simulink model "lo_osc_test"  (Simulink 7.4)
settings: Solver=ode45  StartTime=0.0  StopTime=1000  RelTol=1e-3
libraries: xbsIndex_r4 x8
settings Model: Creator=chenhong  LastModifiedBy=chenhong

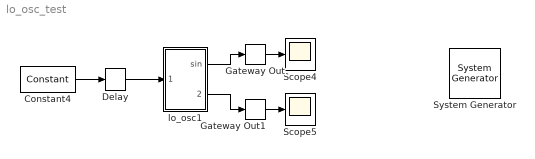
== system lo_osc_test ==
  " System Generator" : xbsIndex_r4/ System Generator  Tag=genX  SystemSampleTime=-1  xilinxfamily=Virtex6  part=xc6vsx315t  speed=-3  package=ff1156  synthesis_tool=XST  clock_wrapper=Clock Enables  directory=./netlist  testbench=off  simulink_period=1  sysclk_period=10  dcm_input_clock_period=10  incr_netlist=off  trim_vbits=Everywhere in SubSystem  dbl_ovrd=According to Block Masks  core_generation=According to Block Masks  run_coregen=off  deprecated_control=off  eval_field=0  block_type=sysgen
      settings: block_version=11.4
  Constant4 : xbsIndex_r4/Constant  arith_type=Boolean  const=1  n_bits=16  bin_pt=14  explicit_period=on  period=1024  equ=P=C  opselect=C  inp2=PCIN>>17  opr=+  inp1=P  carry=CIN  dbl_ovrd=off  block_type=constant
      settings: block_version=11.4
  Delay : xbsIndex_r4/Delay  en=off  latency=25  dbl_ovrd=off  reg_retiming=off  block_type=delay
      settings: block_version=11.4
  Gateway Out : xbsIndex_r4/Gateway Out  hdl_port=on  timing_constraint=None  locs_specified=off  LOCs={}  block_type=gatewayout
      settings: infoedit="Gateway out block.  Converts Xilinx fixed point inputs into ouputs of type Simulink integer, double, or fixed point.<br><br>Hardware notes:  In hardware these blocks become top level output ports or are discarded, depending on how they are configured."  block_version=11.4
  Gateway Out1 : xbsIndex_r4/Gateway Out  hdl_port=on  timing_constraint=None  locs_specified=off  LOCs={}  block_type=gatewayout
      settings: infoedit="Gateway out block.  Converts Xilinx fixed point inputs into ouputs of type Simulink integer, double, or fixed point.<br><br>Hardware notes:  In hardware these blocks become top level output ports or are discarded, depending on how they are configured."  block_version=11.4
  Scope4 : Scope
  Scope5 : Scope
  lo_osc1 : Subsystem  AncestorBlock=xblocks_library_downconverter/lo_osc  mask(lo_osc){n_bits=8, counter_step=5, counter_start=1, counter_width=8, latency=2}
      mask prompts: n_bits "Output Bitwidth"; counter_step "counter step"; counter_start "counter start value"; counter_width "Counter Bitwidth"; latency "Lookup latency"
      mask help:
      | Generates -sin and cos data using a look-up
      | table.
      mask init:
      | config.source=str2func('lo_osc_init_xblock');
      | config.depend=get_dependlist('lo_osc');
      | config.toplevel=gcb;
      | set_param(gcb,'LinkStatus','inactive');
      | xBlock(config, {config.toplevel,...
      |     'n_bits', n_bits, ...
      |     'counter_step', counter_step, ...
      |     'counter_start', counter_start, ...
      |     'counter_width', counter_width, ...
      |     'latency', latency});
      mask Help: eval('xlWeb(''http://casper.berkeley.edu/wiki/Lo_osc'')')
  wires:
  Constant4/1 -> Delay/1
  lo_osc1/1(sin) -> Gateway Out/1
  lo_osc1/2(cos) -> Gateway Out1/1
  Gateway Out1/1 -> Scope5/1
  Gateway Out/1 -> Scope4/1
  Delay/1 -> lo_osc1/1(sync)

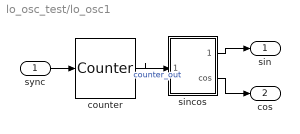
== system lo_osc_test/lo_osc1 ==
  sync : Inport  OutDataType=sfix(16)  OutScaling=2^0
  counter : xbsIndex_r4/Counter  cnt_type=Free Running  cnt_to=Inf  operation=Up  start_count=1  cnt_by_val=5  arith_type=Unsigned  n_bits=8  bin_pt=0  load_pin=off  rst=on  en=off  explicit_period=on  period=1  dbl_ovrd=off  use_behavioral_HDL=off  implementation=Fabric  block_type=counter
      settings: block_version=11.4
  sincos : Subsystem
      settings: AttributesFormatString=|
      | depth_bits = 8
      | bit_width = 8
  sin : Outport  OutDataType=sfix(16)  OutScaling=2^0
  cos : Outport  Port=2  OutDataType=sfix(16)  OutScaling=2^0
  wires:
  sincos/2(cos) -> cos/1
  sincos/1(-sine) -> sin/1
  counter/1 -> sincos/1(theta)  "counter_out"
  sync/1 -> counter/1

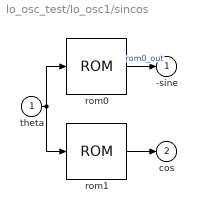
== system lo_osc_test/lo_osc1/sincos ==
  theta : Inport
  rom0 : xbsIndex_r4/ROM  depth=256  initVector=[-0 -0.0245412285229123 -0.049067674327418 -0.0735645635996674 -0.0980171403295606 -0.122410675199216 -0.146730474455362 -0.170961888760301 -0.195090322016128 -0.21910124015687 -0.242980179903264 -0.266712757474898 -0.290284677254462 -0.313681740398892 -0.33688985339222 -0.359895036534988 -0.38268343236509 -0.40524131400499 -0.427555093430282 -0.449611329654607 -0.471396736825998 -0.492898192229784 -0.514102744193222 -0.534997619887097 -0.555570233019602 -0.575808191417845 -0.595699304492433 -0.615231590580627 -0.634393284163645 -0.653172842953777 -0.671558954847018 -0.689540544737067 -0.707106781186547 -0.724247082951467 -0.740951125354959 -0.757208846506485 -0.773010453362737 -0.788346427626606 -0.803207531480645 -0.817584813151584 -0.831469612302545 -0.844853565249707 -0.857728610000272 -0.870086991108711 -0.881921264348355 -0.893224301195515 -0.903989293123443 -0.914209755703531 -0.923879532511287 -0.932992798834739 -0.941544065183021 -0.949528180593037 -0.956940335732209 -0.96377606579544 -0.970031253194544 -0.975702130038529 -0.98078528040323 -0.985277642388941 -0.989176509964781 -0.99247953459871 -0.995184726672197 -0.99729045667869 -0.998795456205172 -0.999698818696204 -1 -0.999698818696204 -0.998795456205172 -0.99729045667869 -0.995184726672197 -0.99247953459871 -0.989176509964781 -0.985277642388941 -0.98078528040323 -0.975702130038529 -0.970031253194544 -0.96377606579544 -0.956940335732209 -0.949528180593037 -0.941544065183021 -0.932992798834739 -0.923879532511287 -0.914209755703531 -0.903989293123443 -0.893224301195515 -0.881921264348355 -0.870086991108711 -0.857728610000272 -0.844853565249707 -0.831469612302545 -0.817584813151584 -0.803207531480645 -0.788346427626606 -0.773010453362737 -0.757208846506485 -0.740951125354959 -0.724247082951467 -0.707106781186548 -0.689540544737067 -0.671558954847019 -0.653172842953777 -0.634393284163645 -0.615231590580627 -0.595699304492433 -0.575808191417845 -0.555570233019602 -0.534997619887097 -0.514102744193222 -0.492898192229784 -0.471396736825998 -0.449611329654607 -0.427555093430282 -0.40524131400499 -0.38268343236509 -0.359895036534988 -0.33688985339222 -0.313681740398891 -0.290284677254462 -0.266712757474898 -0.242980179903264 -0.21910124015687 -0.195090322016129 -0.170961888760301 -0.146730474455362 -0.122410675199216 -0.0980171403295608 -0.0735645635996677 -0.049067674327418 -0.0245412285229123 -1.22464679914735e-16 0.0245412285229121 0.0490676743274177 0.0735645635996675 0.0980171403295606 0.122410675199216 0.146730474455362 0.170961888760301 0.195090322016128 0.21910124015687 0.242980179903264 0.266712757474898 0.290284677254462 0.313681740398891 0.33688985339222 0.359895036534988 0.38268343236509 0.40524131400499 0.427555093430282 0.449611329654607 0.471396736825998 0.492898192229784 0.514102744193222 0.534997619887097 0.555570233019602 0.575808191417845 0.595699304492433 0.615231590580627 0.634393284163645 0.653172842953777 0.671558954847018 0.689540544737067 0.707106781186547 0.724247082951467 0.740951125354959 0.757208846506484 0.773010453362737 0.788346427626606 0.803207531480645 0.817584813151584 0.831469612302545 0.844853565249707 0.857728610000272 0.870086991108711 0.881921264348355 0.893224301195515 0.903989293123443 0.91420975570353 0.923879532511287 0.932992798834739 0.941544065183021 0.949528180593037 0.956940335732209 0.96377606579544 0.970031253194544 0.975702130038528 0.98078528040323 0.985277642388941 0.989176509964781 0.99247953459871 0.995184726672197 0.99729045667869 0.998795456205172 0.999698818696204 1 0.999698818696204 0.998795456205172 0.99729045667869 0.995184726672197 0.99247953459871 0.989176509964781 0.985277642388941 0.98078528040323 0.975702130038529 0.970031253194544 0.96377606579544 0.956940335732209 0.949528180593037 0.941544065183021 0.932992798834739 0.923879532511287 0.914209755703531 0.903989293123443 0.893224301195515 0.881921264348355 0.870086991108711 0.857728610000272 0.844853565249707 0.831469612302545 0.817584813151584 ...(+684 chars)]  distributed_mem=Block RAM  rst=off  init_reg=0  en=off  latency=2  arith_type="Signed  (2's comp)"  n_bits=8  bin_pt=7  dbl_ovrd=off  optimize=Area  use_rpm=on  block_type=sprom
      settings: block_version=11.4
  rom1 : xbsIndex_r4/ROM  depth=256  initVector=[1 0.999698818696204 0.998795456205172 0.99729045667869 0.995184726672197 0.99247953459871 0.989176509964781 0.985277642388941 0.98078528040323 0.975702130038529 0.970031253194544 0.96377606579544 0.956940335732209 0.949528180593037 0.941544065183021 0.932992798834739 0.923879532511287 0.914209755703531 0.903989293123443 0.893224301195515 0.881921264348355 0.870086991108711 0.857728610000272 0.844853565249707 0.831469612302545 0.817584813151584 0.803207531480645 0.788346427626606 0.773010453362737 0.757208846506485 0.740951125354959 0.724247082951467 0.707106781186548 0.689540544737067 0.671558954847018 0.653172842953777 0.634393284163645 0.615231590580627 0.595699304492433 0.575808191417845 0.555570233019602 0.534997619887097 0.514102744193222 0.492898192229784 0.471396736825998 0.449611329654607 0.427555093430282 0.40524131400499 0.38268343236509 0.359895036534988 0.33688985339222 0.313681740398892 0.290284677254462 0.266712757474898 0.242980179903264 0.21910124015687 0.195090322016128 0.170961888760301 0.146730474455362 0.122410675199216 0.0980171403295608 0.0735645635996675 0.0490676743274181 0.0245412285229123 6.12323399573677e-17 -0.0245412285229121 -0.049067674327418 -0.0735645635996673 -0.0980171403295606 -0.122410675199216 -0.146730474455362 -0.170961888760301 -0.195090322016128 -0.21910124015687 -0.242980179903264 -0.266712757474898 -0.290284677254462 -0.313681740398891 -0.33688985339222 -0.359895036534988 -0.38268343236509 -0.40524131400499 -0.427555093430282 -0.449611329654607 -0.471396736825998 -0.492898192229784 -0.514102744193222 -0.534997619887097 -0.555570233019602 -0.575808191417845 -0.595699304492433 -0.615231590580627 -0.634393284163645 -0.653172842953777 -0.671558954847018 -0.689540544737067 -0.707106781186547 -0.724247082951467 -0.740951125354959 -0.757208846506485 -0.773010453362737 -0.788346427626606 -0.803207531480645 -0.817584813151584 -0.831469612302545 -0.844853565249707 -0.857728610000272 -0.870086991108711 -0.881921264348355 -0.893224301195515 -0.903989293123443 -0.914209755703531 -0.923879532511287 -0.932992798834739 -0.941544065183021 -0.949528180593037 -0.956940335732209 -0.96377606579544 -0.970031253194544 -0.975702130038528 -0.98078528040323 -0.985277642388941 -0.989176509964781 -0.99247953459871 -0.995184726672197 -0.99729045667869 -0.998795456205172 -0.999698818696204 -1 -0.999698818696204 -0.998795456205172 -0.99729045667869 -0.995184726672197 -0.99247953459871 -0.989176509964781 -0.985277642388941 -0.98078528040323 -0.975702130038529 -0.970031253194544 -0.96377606579544 -0.956940335732209 -0.949528180593037 -0.941544065183021 -0.932992798834739 -0.923879532511287 -0.914209755703531 -0.903989293123443 -0.893224301195515 -0.881921264348355 -0.870086991108711 -0.857728610000272 -0.844853565249707 -0.831469612302545 -0.817584813151584 -0.803207531480645 -0.788346427626606 -0.773010453362737 -0.757208846506485 -0.740951125354959 -0.724247082951467 -0.707106781186548 -0.689540544737067 -0.671558954847019 -0.653172842953777 -0.634393284163646 -0.615231590580627 -0.595699304492433 -0.575808191417845 -0.555570233019602 -0.534997619887097 -0.514102744193222 -0.492898192229784 -0.471396736825998 -0.449611329654607 -0.427555093430282 -0.40524131400499 -0.38268343236509 -0.359895036534988 -0.33688985339222 -0.313681740398891 -0.290284677254462 -0.266712757474899 -0.242980179903264 -0.21910124015687 -0.195090322016129 -0.170961888760302 -0.146730474455362 -0.122410675199216 -0.0980171403295605 -0.0735645635996674 -0.049067674327418 -0.0245412285229124 -1.83697019872103e-16 0.024541228522912 0.0490676743274177 0.073564563599667 0.0980171403295601 0.122410675199216 0.146730474455362 0.170961888760301 0.195090322016128 0.21910124015687 0.242980179903264 0.266712757474898 0.290284677254462 0.313681740398891 0.33688985339222 0.359895036534988 0.38268343236509 0.40524131400499 0.427555093430282 0.449611329654607 0.471396736825998 0.492898192229784 0.514102744193222 0.534997619887097 0.555570233019602 ...(+697 chars)]  distributed_mem=Block RAM  rst=off  init_reg=0  en=off  latency=2  arith_type="Signed  (2's comp)"  n_bits=8  bin_pt=7  dbl_ovrd=off  optimize=Area  use_rpm=on  block_type=sprom
      settings: block_version=11.4
  -sine : Outport
  cos : Outport  Port=2
  wires:
  theta/1 -> rom1/1, rom0/1
  rom1/1 -> cos/1
  rom0/1 -> -sine/1  "rom0_out"
